simulink model "model_checks"  (R2016b)
settings: Solver=VariableStepAuto  StartTime=0.0  StopTime=20  RelTol=1e-3
values from neighbouring files (symbols this model uses):
  MOT = setup_mot('update', MOT)    [setup_sim.m]
undefined symbols (not defined in the file or in its folder): DiscIntNeverNeededParam
libraries: aerolibutil x1, aerolibtransform2 x1
settings Model: Creator=Andrew  LastModifiedBy=Andrew

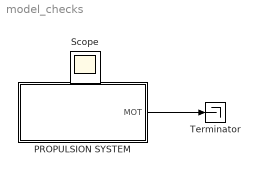
== system model_checks ==
  PROPULSION SYSTEM : Subsystem  AncestorBlock=MOT_lib/PROPULSION SYSTEM
  Terminator : Terminator
  Scope : Scope
  wires:
  PROPULSION SYSTEM/1(MOT) -> Terminator/1

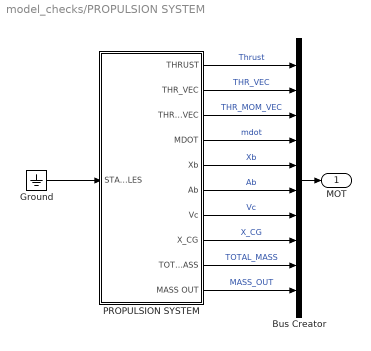
== system model_checks/PROPULSION SYSTEM ==
  Bus Creator : BusCreator  Inputs=10
  Ground : Ground
  PROPULSION SYSTEM : Subsystem
  MOT : Outport
  wires:
  PROPULSION SYSTEM/2(THR_VEC) -> Bus Creator/2  "THR_VEC"
  PROPULSION SYSTEM/3(THR_MOM_VEC) -> Bus Creator/3  "THR_MOM_VEC"
  PROPULSION SYSTEM/9(TOTAL_MASS) -> Bus Creator/9  "TOTAL_MASS"
  PROPULSION SYSTEM/8(X_CG) -> Bus Creator/8  "X_CG"
  PROPULSION SYSTEM/7(Vc) -> Bus Creator/7  "Vc"
  PROPULSION SYSTEM/5(Xb) -> Bus Creator/5  "Xb"
  PROPULSION SYSTEM/10(MASS OUT) -> Bus Creator/10  "MASS_OUT"
  PROPULSION SYSTEM/6(Ab) -> Bus Creator/6  "Ab"
  Bus Creator/1 -> MOT/1
  PROPULSION SYSTEM/4(MDOT) -> Bus Creator/4  "mdot"
  PROPULSION SYSTEM/1(THRUST) -> Bus Creator/1  "Thrust"
  Ground/1 -> PROPULSION SYSTEM/1(STAB_ANGLES)

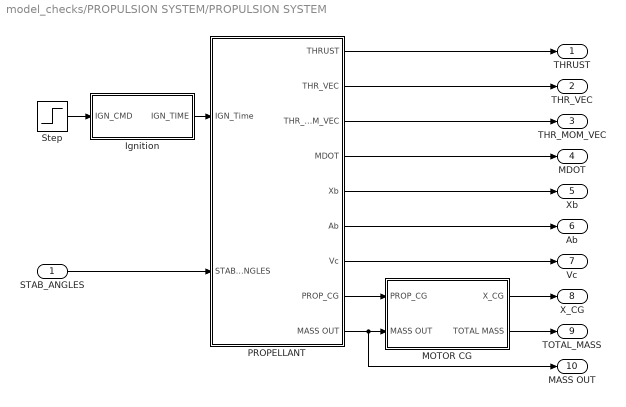
== system model_checks/PROPULSION SYSTEM/PROPULSION SYSTEM ==
  STAB_ANGLES : Inport
  Ignition : Subsystem
  MOTOR CG : Subsystem
  PROPELLANT : Subsystem
  Step : Step  Time=0.005  SampleTime=0
  THRUST : Outport
  THR_VEC : Outport  Port=2
  THR_MOM_VEC : Outport  Port=3
  MDOT : Outport  Port=4
  Xb : Outport  Port=5
  Ab : Outport  Port=6
  Vc : Outport  Port=7
  X_CG : Outport  Port=8
  TOTAL_MASS : Outport  Port=9
  MASS OUT : Outport  Port=10
  wires:
  STAB_ANGLES/1 -> PROPELLANT/2(STAB_ANGLES)
  PROPELLANT/3(THR_MOM_VEC) -> THR_MOM_VEC/1
  PROPELLANT/2(THR_VEC) -> THR_VEC/1
  Step/1 -> Ignition/1(IGN_CMD)
  MOTOR CG/2(TOTAL MASS) -> TOTAL_MASS/1
  MOTOR CG/1(X_CG) -> X_CG/1
  PROPELLANT/8("PROP_CG ") -> MOTOR CG/1(PROP_CG)
  Ignition/1(IGN_TIME) -> PROPELLANT/1(IGN_Time)
  PROPELLANT/7(Vc) -> Vc/1
  PROPELLANT/6(Ab) -> Ab/1
  PROPELLANT/5(Xb) -> Xb/1
  PROPELLANT/9(MASS OUT) -> MASS OUT/1, MOTOR CG/2(MASS OUT)
  PROPELLANT/4(MDOT) -> MDOT/1
  PROPELLANT/1(THRUST) -> THRUST/1

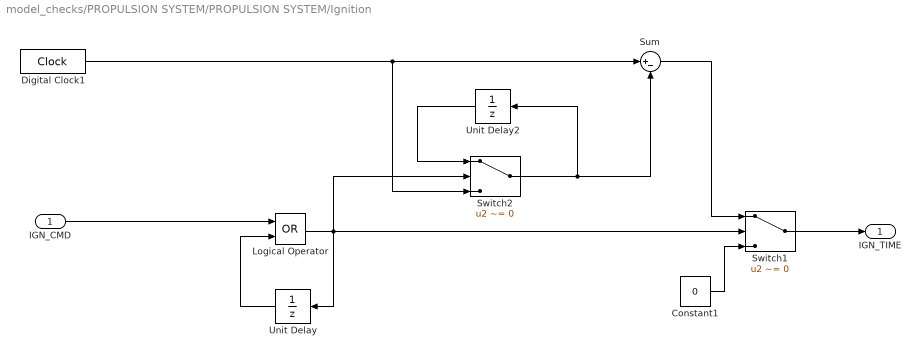
== system model_checks/PROPULSION SYSTEM/PROPULSION SYSTEM/Ignition ==
  IGN_CMD : Inport
  Constant1 : Constant  Value=0
  Digital Clock1 : DigitalClock  SampleTime=0.0025
  Logical Operator : Logic  Operator=OR  AllPortsSameDT=off  OutDataTypeStr=boolean
  Sum : Sum  Inputs=|+-
  Switch1 : Switch  Criteria=u2 ~= 0
  Switch2 : Switch  Criteria=u2 ~= 0
  Unit Delay : UnitDelay  SampleTime=-1
  Unit Delay2 : UnitDelay  SampleTime=-1
  IGN_TIME : Outport
  wires:
  IGN_CMD/1 -> Logical Operator/1
  Unit Delay2/1 -> Switch2/1
  Switch2/1 -> Sum/2, Unit Delay2/1
  Switch1/1 -> IGN_TIME/1
  Sum/1 -> Switch1/1
  Digital Clock1/1 -> Sum/1, Switch2/3
  Logical Operator/1 -> Switch2/2, Unit Delay/1, Switch1/2
  Constant1/1 -> Switch1/3
  Unit Delay/1 -> Logical Operator/2

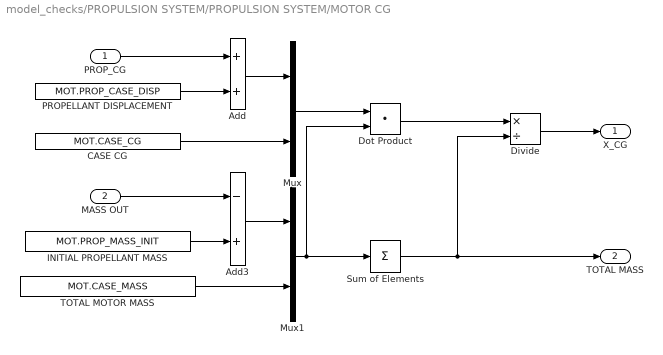
== system model_checks/PROPULSION SYSTEM/PROPULSION SYSTEM/MOTOR CG ==
  PROP_CG : Inport
  MASS OUT : Inport  Port=2
  Add : Sum
  Add3 : Sum  Inputs=-+
  CASE CG : Constant  Value=MOT.CASE_CG
  Divide : Product  Inputs=*/
  Dot Product : DotProduct  InputSameDT=on  OutDataTypeStr=Inherit: Inherit via internal rule
  INITIAL PROPELLANT MASS : Constant  Value=MOT.PROP_MASS_INIT
  Mux : Mux  Inputs=2
  Mux1 : Mux  Inputs=2
  PROPELLANT DISPLACEMENT : Constant  Value=MOT.PROP_CASE_DISP
  Sum of Elements : Sum  Inputs=+
  TOTAL MOTOR MASS : Constant  Value=MOT.CASE_MASS
  X_CG : Outport
  TOTAL MASS : Outport  Port=2
  wires:
  Dot Product/1 -> Divide/1
  Divide/1 -> X_CG/1
  Sum of Elements/1 -> TOTAL MASS/1, Divide/2
  INITIAL PROPELLANT MASS/1 -> Add3/2
  MASS OUT/1 -> Add3/1
  Add3/1 -> Mux1/1
  TOTAL MOTOR MASS/1 -> Mux1/2
  Mux1/1 -> Sum of Elements/1, Dot Product/2
  Mux/1 -> Dot Product/1
  CASE CG/1 -> Mux/2
  Add/1 -> Mux/1
  PROPELLANT DISPLACEMENT/1 -> Add/2
  PROP_CG/1 -> Add/1

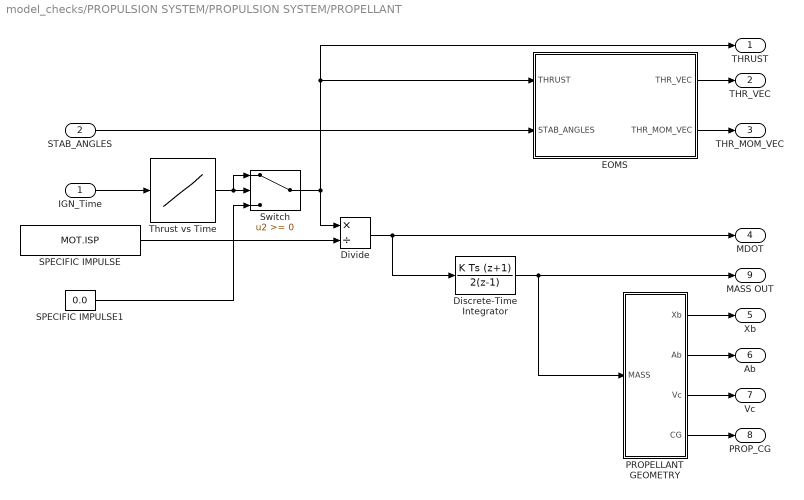
== system model_checks/PROPULSION SYSTEM/PROPULSION SYSTEM/PROPELLANT ==
  IGN_Time : Inport
  STAB_ANGLES : Inport  Port=2
  Discrete-Time Integrator : DiscreteIntegrator  IntegratorMethod=Integration: Trapezoidal  InitialConditionSetting=State (most efficient)  SampleTime=-1  ICPrevOutput=DiscIntNeverNeededParam  ICPrevScaledInput=DiscIntNeverNeededParam
  Divide : Product  Inputs=*/
  EOMS : Subsystem
  PROPELLANT GEOMETRY : Subsystem
  SPECIFIC IMPULSE : Constant  Value=MOT.ISP
  SPECIFIC IMPULSE1 : Constant  Value=0.0
  Switch : Switch
  Thrust vs Time : Lookup_n-D  NumberOfTableDimensions=1  BreakpointsForDimension1=MOT.THRUST_TABLE_X  Table=MOT.THRUST_TABLE_Y  InternalRulePriority=Speed  RndMeth=Simplest  InputSameDT=on
  THRUST : Outport
  THR_VEC : Outport  Port=2
  THR_MOM_VEC : Outport  Port=3
  MDOT : Outport  Port=4
  Xb : Outport  Port=5
  Ab : Outport  Port=6
  Vc : Outport  Port=7
  "PROP_CG " : Outport  Port=8
  MASS OUT : Outport  Port=9
  wires:
  SPECIFIC IMPULSE1/1 -> Switch/3
  Switch/1 -> Divide/1, EOMS/1(THRUST), THRUST/1
  Thrust vs Time/1 -> Switch/1, Switch/2
  STAB_ANGLES/1 -> EOMS/2(STAB_ANGLES)
  EOMS/2(THR_MOM_VEC) -> THR_MOM_VEC/1
  EOMS/1(THR_VEC) -> THR_VEC/1
  Divide/1 -> Discrete-Time Integrator/1, MDOT/1
  SPECIFIC IMPULSE/1 -> Divide/2
  IGN_Time/1 -> Thrust vs Time/1
  PROPELLANT GEOMETRY/1(Xb) -> Xb/1
  PROPELLANT GEOMETRY/4(CG) -> "PROP_CG "/1
  PROPELLANT GEOMETRY/3(Vc) -> Vc/1
  Discrete-Time Integrator/1 -> MASS OUT/1, PROPELLANT GEOMETRY/1(MASS)
  PROPELLANT GEOMETRY/2(Ab) -> Ab/1

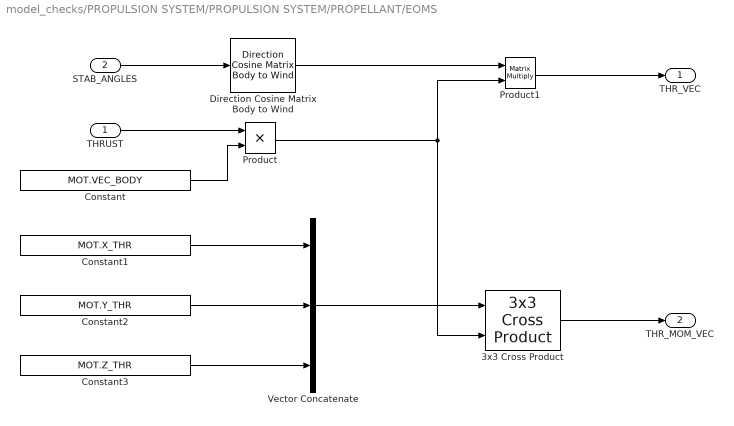
== system model_checks/PROPULSION SYSTEM/PROPULSION SYSTEM/PROPELLANT/EOMS ==
  THRUST : Inport
  STAB_ANGLES : Inport  Port=2
  3x3 Cross Product : aerolibutil/3x3 Cross Product
  Constant : Constant  Value=MOT.VEC_BODY
  Constant1 : Constant  Value=MOT.X_THR
  Constant2 : Constant  Value=MOT.Y_THR
  Constant3 : Constant  Value=MOT.Z_THR
  Direction Cosine Matrix Body to Wind : aerolibtransform2/Direction Cosine Matrix Body to Wind
  Product : Product
  Product1 : Product  Multiplication=Matrix(*)
  Vector Concatenate : Concatenate  NumInputs=3
  THR_VEC : Outport
  THR_MOM_VEC : Outport  Port=2
  wires:
  STAB_ANGLES/1 -> Direction Cosine Matrix Body to Wind/1
  Product1/1 -> THR_VEC/1
  Direction Cosine Matrix Body to Wind/1 -> Product1/1
  3x3 Cross Product/1 -> THR_MOM_VEC/1
  Vector Concatenate/1 -> 3x3 Cross Product/1
  Constant3/1 -> Vector Concatenate/3
  Constant2/1 -> Vector Concatenate/2
  Constant1/1 -> Vector Concatenate/1
  Product/1 -> 3x3 Cross Product/2, Product1/2
  Constant/1 -> Product/2
  THRUST/1 -> Product/1

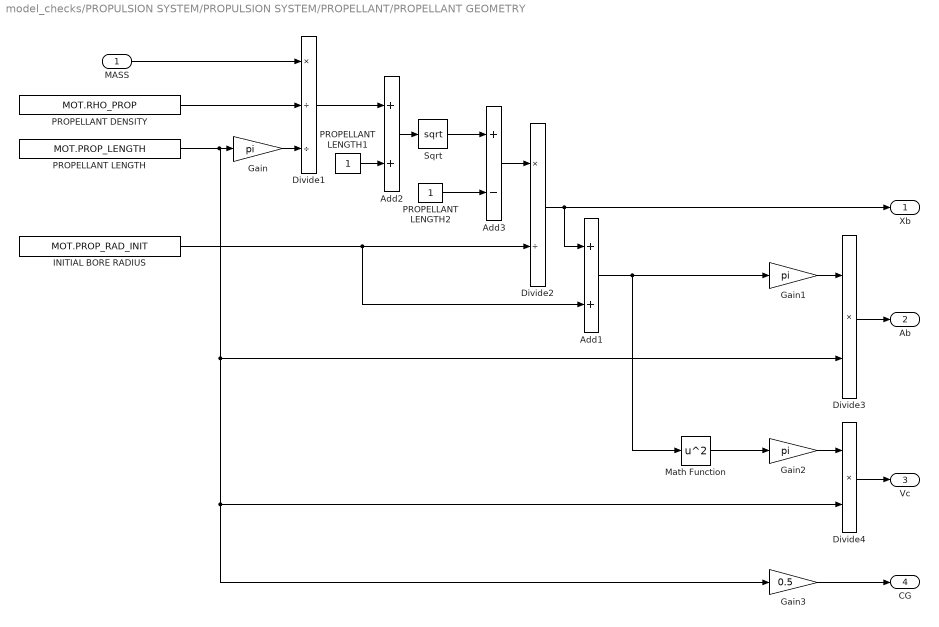
== system model_checks/PROPULSION SYSTEM/PROPULSION SYSTEM/PROPELLANT/PROPELLANT GEOMETRY ==
  MASS : Inport
  Add1 : Sum
  Add2 : Sum
  Add3 : Sum  Inputs=+-
  Divide1 : Product  Inputs=*//
  Divide2 : Product  Inputs=*/
  Divide3 : Product  Inputs=**
  Divide4 : Product  Inputs=**
  Gain : Gain  Gain=pi
  Gain1 : Gain  Gain=pi
  Gain2 : Gain  Gain=pi
  Gain3 : Gain  Gain=0.5
  INITIAL BORE RADIUS : Constant  Value=MOT.PROP_RAD_INIT
  Math Function : Math  Operator=square  SaturateOnIntegerOverflow=on
  PROPELLANT DENSITY : Constant  Value=MOT.RHO_PROP
  PROPELLANT LENGTH : Constant  Value=MOT.PROP_LENGTH
  PROPELLANT LENGTH1 : Constant
  PROPELLANT LENGTH2 : Constant
  Sqrt : Sqrt  SaturateOnIntegerOverflow=on
  Xb : Outport
  Ab : Outport  Port=2
  Vc : Outport  Port=3
  CG : Outport  Port=4
  wires:
  Gain3/1 -> CG/1
  Math Function/1 -> Gain2/1
  Gain2/1 -> Divide4/1
  Divide4/1 -> Vc/1
  Divide3/1 -> Ab/1
  Gain1/1 -> Divide3/1
  Add1/1 -> Math Function/1, Gain1/1
  INITIAL BORE RADIUS/1 -> Divide2/2, Add1/2
  Divide2/1 -> Add1/1, Xb/1
  Add3/1 -> Divide2/1
  MASS/1 -> Divide1/1
  PROPELLANT LENGTH/1 -> Gain/1, Divide4/2, Gain3/1, Divide3/2
  PROPELLANT LENGTH1/1 -> Add2/2
  PROPELLANT LENGTH2/1 -> Add3/2
  Sqrt/1 -> Add3/1
  Add2/1 -> Sqrt/1
  Divide1/1 -> Add2/1
  Gain/1 -> Divide1/3
  PROPELLANT DENSITY/1 -> Divide1/2
